simulink model "SensorFaultInj"  (R2013a)
settings: Solver=FixedStepDiscrete  SolverMode=SingleTasking  StartTime=0.0  StopTime=SimLength  FixedStep=SampleTime  RelTol=1e-3
values from neighbouring files (symbols this model uses):
  GlobalSeed = 10    [start_framework07.m]
  SampleTime = 0.01    [start_framework07.m]
  SimLength = 40    [start_framework07.m]
undefined symbols (not defined in the file or in its folder): DiscIntNeverNeededParam
libraries: dspswit3 x48, simulink x32
(part 3 of 9)

== system SensorFaultInj/FIM_Muster1/occurrence1/flank to dlock2 ==
  flank : Inport
  delay : Inport  Port=2
  Constant : Constant
  Constant1 : Constant  Value=0
  Counter2 : dspswit3/Counter  Direction=Up  CountEvent=Rising edge  CounterSize=User defined  MaxCount=512  InitialCount=0  Output=Count and Hit  HitValue=1  ResetInput=on  SamplesPerFrame=1  Ts=-1  CntDtype=double  HitDtype=Boolean
  Switch : Switch  Criteria=u2 > Threshold
  Variable Time Delay : VariableTransportDelay  MaximumDelay=512  ZeroDelay=on
  conv0 : DataTypeConversion  OutDataTypeStr=boolean
  conv1 : DataTypeConversion  OutDataTypeStr=double
  flag1 : Switch  Threshold=1
  block : Outport
  wires:
  Constant/1 -> flag1/1, Switch/1
  Constant1/1 -> Switch/3, flag1/3
  flank/1 -> Switch/2
  Switch/1 -> Counter2/1
  Counter2/1 -> flag1/2
  delay/1 -> Variable Time Delay/2
  Variable Time Delay/1 -> conv0/1
  flag1/1 -> block/1
  conv0/1 -> Counter2/2
  Counter2/2 -> conv1/1
  conv1/1 -> Variable Time Delay/1

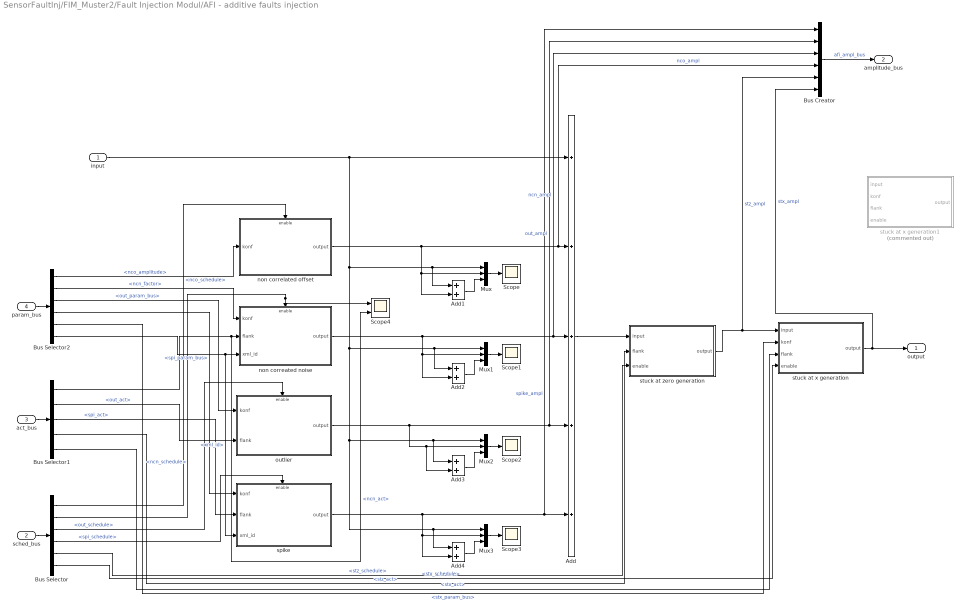
== system SensorFaultInj/FIM_Muster2/Fault Injection Modul/AFI - additive faults injection ==
  input : Inport
  sched_bus : Inport  Port=2
  act_bus : Inport  Port=3
  param_bus : Inport  Port=4
  Add : Sum  Inputs=+++++
  Add{1..4} (4 alike) : Sum
  Bus Creator : BusCreator  Inputs=6
  Bus Selector : BusSelector  OutputSignals=nco_schedule,ncn_schedule,out_schedule,spi_schedule,stz_schedule,stx_schedule
  Bus Selector1 : BusSelector  OutputSignals=ncn_act,out_act,spi_act,stz_act,stx_act
  Bus Selector2 : BusSelector  OutputSignals=nco_amplitude,ncn_factor,out_param_bus,spi_param_bus,stx_param_bus,xml_id
  Mux{,1..3} (4 alike) : Mux  Inputs=3
  Scope{,1..3} (4 alike) : Scope
      Scope settings: YMin=-70  YMax=70  SaveName=ScopeData14  MaxDataPoints=10000
      Scope1 settings: YMin=-50  YMax=55  SaveName=ScopeData15
      Scope2 settings: YMin=-70  YMax=70  SaveName=ScopeData16
      Scope3 settings: YMin=-50  YMax=60  SaveName=ScopeData17
  Scope4 : Scope  NumInputPorts=2
      settings: YMin=-70~-5  YMax=70~5  SaveName=ScopeData28
  non correated noise : Subsystem
  non correlated offset : Subsystem
  outlier : Subsystem
  spike : Subsystem
  stuck at x generation : Subsystem
  stuck at x generation1 : Subsystem  Commented=on
  stuck at zero generation : Subsystem
  output : Outport
  "amplitude_bus " : Outport  Port=2
  wires:
  input/1 -> Add1/1, Mux/1, Add4/1, Mux3/1, Add3/1, Mux2/1, Add2/1, Mux1/1, Add/1
  non correlated offset/1(output) -> Add1/2, Mux/2, Bus Creator/4, Add/2  "nco_ampl"
  non correated noise/1(output) -> Add2/2, Mux1/2, Bus Creator/3, Add/3  "ncn_ampl"
  outlier/1(output) -> Add3/2, Mux2/2, Bus Creator/2, Add/4  "out_ampl"
  spike/1(output) -> Bus Creator/1, Add/5, Add4/2, Mux3/2  "spike_ampl"
  Mux/1 -> Scope/1
  Mux1/1 -> Scope1/1
  Mux2/1 -> Scope2/1
  Mux3/1 -> Scope3/1
  Add1/1 -> Mux/3
  Add2/1 -> Mux1/3
  Add3/1 -> Mux2/3
  Add4/1 -> Mux3/3
  Add/1 -> stuck at zero generation/1(input)
  stuck at x generation/1(output) -> Bus Creator/6, output/1  "stx_ampl"
  stuck at zero generation/1(output) -> Bus Creator/5, stuck at x generation/1(input)  "stz_ampl"
  sched_bus/1 -> Bus Selector/1
  Bus Selector/1 -> non correlated offset/Enable  "<nco_schedule>"
  Bus Selector/2 -> Scope4/1, non correated noise/Enable  "<ncn_schedule>"
  Bus Selector/5 -> stuck at zero generation/3(enable)  "<stz_schedule>"
  Bus Selector/6 -> stuck at x generation/4(enable)  "<stx_schedule>"
  act_bus/1 -> Bus Selector1/1
  Bus Selector1/1 -> Scope4/2, non correated noise/2(flank)  "<ncn_act>"
  Bus Selector1/2 -> outlier/2(flank)  "<out_act>"
  Bus Selector1/3 -> spike/2(flank)  "<spi_act>"
  Bus Selector1/4 -> stuck at zero generation/2(flank)  "<stz_act>"
  Bus Selector1/5 -> stuck at x generation/3(flank)  "<stx_act>"
  param_bus/1 -> Bus Selector2/1
  Bus Selector2/1 -> non correlated offset/1(konf)  "<nco_amplitude>"
  Bus Selector2/2 -> non correated noise/1("konf ")  "<ncn_factor>"
  Bus Selector2/3 -> outlier/1(konf)  "<out_param_bus>"
  Bus Selector2/4 -> spike/1(konf)  "<spi_param_bus>"
  Bus Selector2/5 -> stuck at x generation/2(konf)  "<stx_param_bus>"
  Bus Selector2/6 -> spike/3(xml_id), non correated noise/3(xml_id)  "<xml_id>"
  Bus Creator/1 -> "amplitude_bus "/1  "afi_ampl_bus"
  Bus Selector/3 -> outlier/Enable  "<out_schedule>"
  Bus Selector/4 -> spike/Enable  "<spi_schedule>"

== system SensorFaultInj/FIM_Muster2/Fault Injection Modul/FFI - functional fault injection ==
  input : Inport
  schedule_port : Inport  Port=2
  param_port : Inport  Port=3
  Bus Creator : BusCreator  Inputs=3
  Bus Selector : BusSelector  OutputSignals=sat_schedule,ncd_schedule,tcd_schedule
  Bus Selector1 : BusSelector  OutputSignals=sat_param_bus,ncd_delay,tcd_delay,xml_id
  Mux1 : Mux  Inputs=2
  Mux3 : Mux  Inputs=3
  Scope3 : Scope  NumInputPorts=2
      settings: YMin=-50~-50  YMax=50~50  SaveName=ScopeData6
  "const delay " : Subsystem
  saturation : Subsystem
  "time correlated delay " : Subsystem
  output : Outport
  amplitude_port : Outport  Port=2
  wires:
  input/1 -> Mux3/1, Mux1/1, saturation/1(input)
  Mux1/1 -> Scope3/1
  Mux3/1 -> Scope3/2
  saturation/1(output) -> Mux1/2, Bus Creator/1, "const delay "/1(input)  "sat_ampl"
  "const delay "/1(output1) -> "time correlated delay "/1(input), Mux3/2
  "time correlated delay "/1(output1) -> Mux3/3, output/1
  schedule_port/1 -> Bus Selector/1
  param_port/1 -> Bus Selector1/1
  Bus Selector1/4 -> "time correlated delay "/4(xml id)  "<xml_id>"
  Bus Selector1/3 -> "time correlated delay "/2(konf)  "<tcd_delay>"
  Bus Selector1/1 -> saturation/2("konf ")  "<sat_param_bus>"
  Bus Selector1/2 -> "const delay "/2(konf)  "<ncd_delay>"
  Bus Selector/1 -> saturation/3(enable)  "<sat_schedule>"
  Bus Selector/2 -> "const delay "/3(enable)  "<ncd_schedule>"
  Bus Selector/3 -> "time correlated delay "/3(enable)  "<tcd_schedule>"
  Bus Creator/1 -> amplitude_port/1  "ffi_ampl_bus"
  "const delay "/2(delay) -> Bus Creator/2  "ncd_ampl"
  "time correlated delay "/2(delay) -> Bus Creator/3  "tcd_ampl"

== system SensorFaultInj/FIM_Muster2/Fault Injection Modul/MFI - multiplicative fault injection ==
  In1 : Inport
  sched_port : Inport  Port=2
  act_port : Inport  Port=3
  param_port : Inport  Port=4
  Add : Sum  Inputs=+++++
  Add{1..4} (4 alike) : Sum
  Bus Creator : BusCreator
  Bus Selector : BusSelector  OutputSignals=vco_schedule,tco_schedule,vcn_schedule,tcn_schedule
  Bus Selector1 : BusSelector  OutputSignals=vcn_act,tcn_act
  Bus Selector2 : BusSelector  OutputSignals=vco_factor,tco_amplitude,vcn_factor,tcn_factor,xml_id
  Mux{,1..3} (4 alike) : Mux  Inputs=3
  Scope{,1..3} (4 alike) : Scope
      Scope settings: YMin=-55  YMax=55  SaveName=ScopeData8
      Scope1 settings: YMin=-50  YMax=55  SaveName=ScopeData11  MaxDataPoints=10000
      Scope2 settings: YMin=-70  YMax=70  SaveName=ScopeData12
      Scope3 settings: YMin=-50  YMax=60  SaveName=ScopeData13
  time correlated noise : Subsystem  TreatAsAtomicUnit=on
  time correlated offset : Subsystem  TreatAsAtomicUnit=on
  value correlated noise : Subsystem
  value correlated offset : Subsystem  TreatAsAtomicUnit=on
  output : Outport
  "amplitude_port " : Outport  Port=2
  wires:
  In1/1 -> Mux3/1, Add4/1, Mux2/1, Add3/1, Mux1/1, Add2/1, Mux/1, Add1/1, Add/1, value correlated noise/1(input), value correlated offset/1(input)
  value correlated offset/1(output) -> Bus Creator/4, Add/2, Add1/2, Mux/2  "vco_ampl"
  time correlated offset/1(output) -> Add2/2, Mux1/2, Bus Creator/3, Add/3  "tco_ampl"
  value correlated noise/1(output) -> Add3/2, Mux2/2, Bus Creator/2, Add/4  "vcn_ampl"
  time correlated noise/1(output) -> Add4/2, Mux3/2, Bus Creator/1, Add/5  "tcn_ampl"
  Mux/1 -> Scope/1
  Mux1/1 -> Scope1/1
  Mux2/1 -> Scope2/1
  Mux3/1 -> Scope3/1
  Add1/1 -> Mux/3
  Add2/1 -> Mux1/3
  Add3/1 -> Mux2/3
  Add4/1 -> Mux3/3
  Add/1 -> output/1
  sched_port/1 -> Bus Selector/1
  Bus Selector/1 -> value correlated offset/Enable  "<vco_schedule>"
  Bus Selector/2 -> time correlated offset/Enable  "<tco_schedule>"
  Bus Selector/3 -> value correlated noise/Enable  "<vcn_schedule>"
  Bus Selector/4 -> time correlated noise/Enable  "<tcn_schedule>"
  act_port/1 -> Bus Selector1/1
  Bus Selector1/2 -> time correlated noise/2(flank)  "<tcn_act>"
  Bus Selector1/1 -> value correlated noise/3(flank)  "<vcn_act>"
  param_port/1 -> Bus Selector2/1
  Bus Selector2/5 -> value correlated noise/4(xml_id), time correlated noise/3(xml id), time correlated offset/2(xml id)  "<xml_id>"
  Bus Selector2/1 -> value correlated offset/2(konf)  "<vco_factor>"
  Bus Selector2/2 -> time correlated offset/1(konf)  "<tco_amplitude>"
  Bus Selector2/3 -> value correlated noise/2(konf)  "<vcn_factor>"
  Bus Selector2/4 -> time correlated noise/1(konf)  "<tcn_factor>"
  Bus Creator/1 -> "amplitude_port "/1  "mfi_amp_bus"

== system SensorFaultInj/FIM_Muster2/Fault Injection Modul/activation bus creator ==
  act_port : Inport
  Bus Selector : BusSelector  OutputSignals=vcn_act,tcn_act  OutputAsBus=on
  Bus Selector1 : BusSelector  OutputSignals=ncn_act,out_act,spi_act,stz_act,stx_act  OutputAsBus=on
  mfi_act_port : Outport
  afi_act_port : Outport  Port=2
  wires:
  act_port/1 -> Bus Selector1/1, Bus Selector/1
  Bus Selector/1 -> mfi_act_port/1  "mfi_act_bus"
  Bus Selector1/1 -> afi_act_port/1  "afi_act_bus"

== system SensorFaultInj/FIM_Muster2/Fault Injection Modul/schedule bus creator ==
  schedule_port : Inport
  Bus Selector : BusSelector  OutputSignals=vco_schedule,tco_schedule,vcn_schedule,tcn_schedule  OutputAsBus=on
  Bus Selector1 : BusSelector  OutputSignals=nco_schedule,ncn_schedule,spi_schedule,out_schedule,stz_schedule,stx_schedule  OutputAsBus=on
  Bus Selector2 : BusSelector  OutputSignals=sat_schedule,ncd_schedule,tcd_schedule  OutputAsBus=on
  mfi_sched_port : Outport
  afi_sched_port : Outport  Port=2
  ffi_sched_port : Outport  Port=3
  wires:
  schedule_port/1 -> Bus Selector2/1, Bus Selector1/1, Bus Selector/1
  Bus Selector/1 -> mfi_sched_port/1  "mfi_sched_bus"
  Bus Selector1/1 -> afi_sched_port/1  "afi_sched_bus"
  Bus Selector2/1 -> ffi_sched_port/1  "ffi_sched_bus"

== system SensorFaultInj/FIM_Muster2/Fault Injection Modul/schedule bus creator1 ==
  schedule_port : Inport
  Bus Selector : BusSelector  OutputSignals=parameter_bus.vco_factor,parameter_bus.tco_amplitude,parameter_bus.vcn_factor,parameter_bus.tcn_factor,xml_id  OutputAsBus=on
  Bus Selector1 : BusSelector  OutputSignals=parameter_bus.nco_amplitude,parameter_bus.ncn_factor,parameter_bus.out_param_bus,parameter_bus.spi_param_bus,parameter_bus.stx_param_bus,xml_id  OutputAsBus=on
  Bus Selector2 : BusSelector  OutputSignals=parameter_bus.sat_param_bus,parameter_bus.ncd_delay,parameter_bus.tcd_delay,xml_id  OutputAsBus=on
  mfi_sched_port : Outport
  afi_sched_port : Outport  Port=2
  ffi_sched_port : Outport  Port=3
  wires:
  schedule_port/1 -> Bus Selector2/1, Bus Selector1/1, Bus Selector/1
  Bus Selector/1 -> mfi_sched_port/1  "mfi_sched_bus"
  Bus Selector1/1 -> afi_sched_port/1  "afi_sched_bus"
  Bus Selector2/1 -> ffi_sched_port/1  "ffi_sched_bus"

== system SensorFaultInj/FIM_Muster2/Parser Modul/occurence parser  ==
  In1 : Inport
  Add1 : Sum
  Constant1 : Constant
  Digital Clock2 : DigitalClock  SampleTime=SampleTime
  Enabled Subsystem : Subsystem  TreatAsAtomicUnit=on
  Memory2 : Memory
  Subtract2 : Sum  Inputs=+-
  Out1 : Outport
  wires:
  Digital Clock2/1 -> Add1/2
  Memory2/1 -> Subtract2/2
  Constant1/1 -> Add1/1, Subtract2/1
  Add1/1 -> Memory2/1
  Subtract2/1 -> Enabled Subsystem/Enable
  Enabled Subsystem/1(Out1) -> Out1/1
  In1/1 -> Enabled Subsystem/1(In1)

== system SensorFaultInj/FIM_Muster2/Parser Modul/parameter parser ==
  In1 : Inport
  Add1 : Sum
  Constant1 : Constant
  Digital Clock2 : DigitalClock  SampleTime=SampleTime
  Enabled Subsystem : Subsystem  TreatAsAtomicUnit=on
  Memory2 : Memory
  Subtract2 : Sum  Inputs=+-
  Out1 : Outport
  wires:
  Digital Clock2/1 -> Add1/2
  Memory2/1 -> Subtract2/2
  Constant1/1 -> Add1/1, Subtract2/1
  Add1/1 -> Memory2/1
  Subtract2/1 -> Enabled Subsystem/Enable
  In1/1 -> Enabled Subsystem/1(In1)
  Enabled Subsystem/1(Out1) -> Out1/1

== system SensorFaultInj/FIM_Muster2/Parser Modul/schedule once per sample step  ==
  In1 : Inport
  Bus Creator : BusCreator  Inputs=13
  schedule_fcn id 0 : Subsystem
  schedule_fcn id 1 : Subsystem
  schedule_fcn id 10 : Subsystem
  schedule_fcn id 11 : Subsystem
  schedule_fcn id 12 : Subsystem
  schedule_fcn id 2 : Subsystem
  schedule_fcn id 3 : Subsystem
  schedule_fcn id 4 : Subsystem
  schedule_fcn id 5 : Subsystem
  schedule_fcn id 6 : Subsystem
  schedule_fcn id 7 : Subsystem
  schedule_fcn id 8 : Subsystem
  schedule_fcn id 9 : Subsystem
  Out1 : Outport
  wires:
  schedule_fcn id 3/1(output) -> Bus Creator/4
  schedule_fcn id 6/1(output) -> Bus Creator/7
  schedule_fcn id 4/1(output) -> Bus Creator/5
  schedule_fcn id 1/1(output) -> Bus Creator/2
  schedule_fcn id 0/1(output) -> Bus Creator/1
  schedule_fcn id 10/1(output) -> Bus Creator/11
  schedule_fcn id 5/1(output) -> Bus Creator/6
  schedule_fcn id 9/1(output) -> Bus Creator/10
  schedule_fcn id 8/1(output) -> Bus Creator/9
  schedule_fcn id 7/1(output) -> Bus Creator/8
  schedule_fcn id 12/1(output) -> Bus Creator/13
  schedule_fcn id 11/1(output) -> Bus Creator/12
  schedule_fcn id 2/1(output) -> Bus Creator/3
  Bus Creator/1 -> Out1/1  "schedule_bus"
  In1/1 -> schedule_fcn id 5/1(In1), schedule_fcn id 4/1(In1), schedule_fcn id 3/1(In1), schedule_fcn id 2/1(In1), schedule_fcn id 1/1(In1), schedule_fcn id 0/1(In1), schedule_fcn id 6/1(In1), schedule_fcn id 7/1(In1), schedule_fcn id 8/1(In1), schedule_fcn id 9/1(In1), schedule_fcn id 10/1(In1), schedule_fcn id 12/1(In1), schedule_fcn id 11/1(In1)

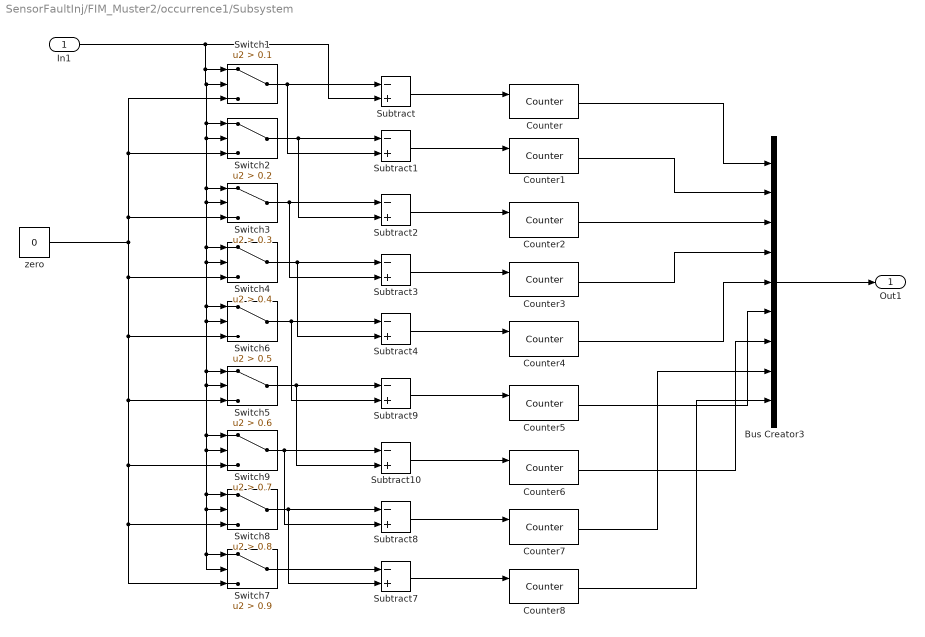
== system SensorFaultInj/FIM_Muster2/occurrence1/Subsystem ==
  In1 : Inport
  Bus Creator3 : BusCreator  Inputs=9
  Counter{,1..8} (9 alike) : dspswit3/Counter  Direction=Up  CountEvent=Non-zero sample  CounterSize=User defined  MaxCount=10000  InitialCount=0  Output=Count  HitValue=32  ResetInput=on  SamplesPerFrame=1  Ts=1  CntDtype=double  HitDtype=Logical
  Subtract{,1..4,7..10} (9 alike) : Sum  Inputs=-+
  Switch1 : Switch  Criteria=u2 > Threshold  Threshold=0.1
  Switch2 : Switch  Criteria=u2 > Threshold  Threshold=0.2
  Switch3 : Switch  Criteria=u2 > Threshold  Threshold=0.3
  Switch4 : Switch  Criteria=u2 > Threshold  Threshold=0.4
  Switch5 : Switch  Criteria=u2 > Threshold  Threshold=0.6
  Switch6 : Switch  Criteria=u2 > Threshold  Threshold=0.5
  Switch7 : Switch  Criteria=u2 > Threshold  Threshold=0.9
  Switch8 : Switch  Criteria=u2 > Threshold  Threshold=0.8
  Switch9 : Switch  Criteria=u2 > Threshold  Threshold=0.7
  zero : Constant  Value=0  OutDataTypeStr=boolean
  Out1 : Outport
  wires:
  Switch1/1 -> Subtract1/2, Subtract/1
  Switch2/1 -> Subtract2/2, Subtract1/1
  Switch3/1 -> Subtract3/2, Subtract2/1
  Switch4/1 -> Subtract4/2, Subtract3/1
  Switch6/1 -> Subtract9/2, Subtract4/1
  Switch5/1 -> Subtract10/2, Subtract9/1
  Switch9/1 -> Subtract8/2, Subtract10/1
  Switch8/1 -> Subtract7/2, Subtract8/1
  Switch7/1 -> Subtract7/1
  Subtract/1 -> Counter/1
  Subtract1/1 -> Counter1/1
  Subtract2/1 -> Counter2/1
  Subtract3/1 -> Counter3/1
  Subtract4/1 -> Counter4/1
  Subtract9/1 -> Counter5/1
  Subtract10/1 -> Counter6/1
  Subtract8/1 -> Counter7/1
  Counter2/1 -> Bus Creator3/3
  Counter3/1 -> Bus Creator3/4
  Counter1/1 -> Bus Creator3/2
  Counter/1 -> Bus Creator3/1
  Counter4/1 -> Bus Creator3/5
  Counter5/1 -> Bus Creator3/6
  Counter6/1 -> Bus Creator3/7
  Counter7/1 -> Bus Creator3/8
  Counter8/1 -> Bus Creator3/9
  Bus Creator3/1 -> Out1/1
  In1/1 -> Switch2/1, Switch3/1, Switch3/2, Switch4/1, Switch4/2, Switch6/1, Switch5/1, Switch9/1, Switch8/1, Switch7/1, Switch7/2, Switch8/2, Switch9/2, Switch5/2, Switch6/2, Switch2/2, Switch1/2, Switch1/1, Subtract/2
  zero/1 -> Switch4/3, Switch6/3, Switch5/3, Switch9/3, Switch7/3, Switch8/3, Switch1/3, Switch2/3, Switch3/3
  Subtract7/1 -> Counter8/1

== system SensorFaultInj/FIM_Muster2/occurrence1/bus_counter ==
  In1 : Inport
  Bus Creator : BusCreator  Inputs=7
  Bus Selector : BusSelector  OutputSignals=vcn_act,tcn_act,ncn_act,out_act,spi_act,stz_act,stx_act
  Counter{,1..3} (4 alike) : dspswit3/Counter  Direction=Up  CountEvent=Non-zero sample  CounterSize=User defined  MaxCount=10000  InitialCount=0  Output=Count  HitValue=32  ResetInput=on  SamplesPerFrame=1  Ts=1  CntDtype=double  HitDtype=Logical
  Counter4 : dspswit3/Counter  Direction=Up  CountEvent=Rising edge  CounterSize=User defined  MaxCount=10000  InitialCount=0  Output=Count  HitValue=32  ResetInput=on  SamplesPerFrame=1  Ts=1  CntDtype=double  HitDtype=Logical
  Counter5 : dspswit3/Counter  Direction=Up  CountEvent=Rising edge  CounterSize=User defined  MaxCount=10000  InitialCount=0  Output=Count  HitValue=32  ResetInput=on  SamplesPerFrame=1  Ts=1  CntDtype=double  HitDtype=Logical
  Counter6 : dspswit3/Counter  Direction=Up  CountEvent=Rising edge  CounterSize=User defined  MaxCount=10000  InitialCount=0  Output=Count  HitValue=32  ResetInput=on  SamplesPerFrame=1  Ts=1  CntDtype=double  HitDtype=Logical
  Out1 : Outport
  wires:
  In1/1 -> Bus Selector/1
  Bus Selector/1 -> Counter/1  "<vcn_act>"
  Counter/1 -> Bus Creator/1
  Counter1/1 -> Bus Creator/2
  Bus Selector/2 -> Counter1/1  "<tcn_act>"
  Bus Selector/3 -> Counter2/1  "<ncn_act>"
  Bus Selector/4 -> Counter3/1  "<out_act>"
  Bus Selector/5 -> Counter4/1  "<spi_act>"
  Bus Selector/6 -> Counter5/1  "<stz_act>"
  Bus Selector/7 -> Counter6/1  "<stx_act>"
  Counter3/1 -> Bus Creator/4
  Counter4/1 -> Bus Creator/5
  Counter6/1 -> Bus Creator/7
  Counter5/1 -> Bus Creator/6
  Counter2/1 -> Bus Creator/3
  Bus Creator/1 -> Out1/1

== system SensorFaultInj/FIM_Muster2/occurrence1/disable non active trigger ==
  vec_probability : Inport
  vec_activation : Inport  Port=2
  Bus Creator : BusCreator  Inputs=7
  Bus Selector : BusSelector  OutputSignals=vcn_occ,tcn_occ,ncn_occ,out_occ,spi_occ,stz_occ,stx_occ
  Bus Selector1 : BusSelector  OutputSignals=vcn_schedule,tcn_schedule,ncn_schedule,out_schedule,spi_schedule,stz_schedule,stx_schedule
  Constant : Constant  Value=0
  Switch{,1..6} (7 alike) : Switch  Threshold=1
  vec_probability_ad : Outport
  wires:
  vec_probability/1 -> Bus Selector/1
  vec_activation/1 -> Bus Selector1/1
  Bus Selector1/1 -> Switch/2  "<vcn_schedule>"
  Bus Selector1/2 -> Switch1/2  "<tcn_schedule>"
  Bus Selector1/3 -> Switch2/2  "<ncn_schedule>"
  Bus Selector1/4 -> Switch3/2  "<out_schedule>"
  Bus Selector1/5 -> Switch6/2  "<spi_schedule>"
  Bus Selector1/6 -> Switch5/2  "<stz_schedule>"
  Bus Selector1/7 -> Switch4/2  "<stx_schedule>"
  Bus Selector/1 -> Switch/1  "<vcn_occ>"
  Bus Selector/2 -> Switch1/1  "<tcn_occ>"
  Bus Selector/3 -> Switch2/1  "<ncn_occ>"
  Bus Selector/4 -> Switch3/1  "<out_occ>"
  Bus Selector/5 -> Switch6/1  "<spi_occ>"
  Constant/1 -> Switch4/3, Switch5/3, Switch6/3, Switch3/3, Switch2/3, Switch1/3, Switch/3
  Switch/1 -> Bus Creator/1  "vcn_occ"
  Switch1/1 -> Bus Creator/2  "tcn_occ"
  Switch2/1 -> Bus Creator/3  "ncn_occ"
  Switch3/1 -> Bus Creator/4  "out_occ"
  Switch6/1 -> Bus Creator/5  "spi_occ"
  Switch5/1 -> Bus Creator/6  "stz_occ"
  Switch4/1 -> Bus Creator/7  "stx_occ"
  Bus Selector/7 -> Switch4/1  "<stx_occ>"
  Bus Selector/6 -> Switch5/1  "<stz_occ>"
  Bus Creator/1 -> vec_probability_ad/1

== system SensorFaultInj/FIM_Muster2/occurrence1/flank to dlock0 ==
  flank : Inport
  delay : Inport  Port=2
  Constant : Constant
  Constant1 : Constant  Value=0
  Counter2 : dspswit3/Counter  Direction=Up  CountEvent=Rising edge  CounterSize=User defined  MaxCount=512  InitialCount=0  Output=Count and Hit  HitValue=1  ResetInput=on  SamplesPerFrame=1  Ts=-1  CntDtype=double  HitDtype=Boolean
  Switch : Switch  Criteria=u2 > Threshold
  Variable Time Delay : VariableTransportDelay  MaximumDelay=512  ZeroDelay=on
  conv0 : DataTypeConversion  OutDataTypeStr=boolean
  conv1 : DataTypeConversion  OutDataTypeStr=double
  flag1 : Switch  Threshold=1
  block : Outport
  wires:
  Constant/1 -> flag1/1, Switch/1
  Constant1/1 -> Switch/3, flag1/3
  flank/1 -> Switch/2
  Switch/1 -> Counter2/1
  Counter2/1 -> flag1/2
  delay/1 -> Variable Time Delay/2
  Variable Time Delay/1 -> conv0/1
  flag1/1 -> block/1
  conv0/1 -> Counter2/2
  Counter2/2 -> conv1/1
  conv1/1 -> Variable Time Delay/1

== system SensorFaultInj/FIM_Muster2/occurrence1/flank to dlock1 ==
  flank : Inport
  delay : Inport  Port=2
  Constant : Constant
  Constant1 : Constant  Value=0
  Counter2 : dspswit3/Counter  Direction=Up  CountEvent=Rising edge  CounterSize=User defined  MaxCount=512  InitialCount=0  Output=Count and Hit  HitValue=1  ResetInput=on  SamplesPerFrame=1  Ts=-1  CntDtype=double  HitDtype=Boolean
  Switch : Switch  Criteria=u2 > Threshold
  Variable Time Delay : VariableTransportDelay  MaximumDelay=512  ZeroDelay=on
  conv0 : DataTypeConversion  OutDataTypeStr=boolean
  conv1 : DataTypeConversion  OutDataTypeStr=double
  flag1 : Switch  Threshold=1
  block : Outport
  wires:
  Constant/1 -> flag1/1, Switch/1
  Constant1/1 -> Switch/3, flag1/3
  flank/1 -> Switch/2
  Switch/1 -> Counter2/1
  Counter2/1 -> flag1/2
  delay/1 -> Variable Time Delay/2
  Variable Time Delay/1 -> conv0/1
  flag1/1 -> block/1
  conv0/1 -> Counter2/2
  Counter2/2 -> conv1/1
  conv1/1 -> Variable Time Delay/1

== system SensorFaultInj/FIM_Muster2/occurrence1/flank to dlock2 ==
  flank : Inport
  delay : Inport  Port=2
  Constant : Constant
  Constant1 : Constant  Value=0
  Counter2 : dspswit3/Counter  Direction=Up  CountEvent=Rising edge  CounterSize=User defined  MaxCount=512  InitialCount=0  Output=Count and Hit  HitValue=1  ResetInput=on  SamplesPerFrame=1  Ts=-1  CntDtype=double  HitDtype=Boolean
  Switch : Switch  Criteria=u2 > Threshold
  Variable Time Delay : VariableTransportDelay  MaximumDelay=512  ZeroDelay=on
  conv0 : DataTypeConversion  OutDataTypeStr=boolean
  conv1 : DataTypeConversion  OutDataTypeStr=double
  flag1 : Switch  Threshold=1
  block : Outport
  wires:
  Constant/1 -> flag1/1, Switch/1
  Constant1/1 -> Switch/3, flag1/3
  flank/1 -> Switch/2
  Switch/1 -> Counter2/1
  Counter2/1 -> flag1/2
  delay/1 -> Variable Time Delay/2
  Variable Time Delay/1 -> conv0/1
  flag1/1 -> block/1
  conv0/1 -> Counter2/2
  Counter2/2 -> conv1/1
  conv1/1 -> Variable Time Delay/1

== system SensorFaultInj/Glogal Activation Generator/Enabled Subsystem/global parser2 ==
  ex_sfun_globalocc : S-Function  FunctionName=ex_sfun_globalocc  EnableBusSupport=off  mask(Legacy Function){SFunctionSpec=double y1 = global_occ(single u1), ShowSpec=on}
      mask prompts: ShowSpec "Display function specification"
      mask help:
      | This block allows you to call the legacy functions specified by the following Legacy Code Tool definition:
      | def.SFunctionName = 'ex_sfun_globalocc';
      | def.OutputFcnSpec = 'double y1 = global_occ(single u1)';
      | def.HeaderFiles = {'global_occ.hpp'};
      | def.SourceFiles = {'global_occ.cpp'};
      | def.Options.language = 'C++';
      mask Help: <p>This block was generated automatically by the Legacy Code Tool. For detailed help on this tool, call<a href="matlab:legacy_code('help')"> legacy_code('help')</a>.</p>
      mask Callback ShowSpec:
      | if strcmp(get_param(gcbh, 'ShowSpec'), 'on')
      |   set_param(gcbh, 'MaskDisplay', sprintf('fprintf(''%s'');', get_param(gcbh, 'SFunctionSpec')));
      | else
      |   set_param(gcbh, 'MaskDisplay', sprintf('fprintf(''%s'');', get_param(gcbh, 'FunctionName')));
      | end
      mask Display: fprintf('double y1 = global_occ(single u1)');
  fault id : Constant  Value=2  OutDataTypeStr=single
  occ : Outport
  wires:
  ex_sfun_globalocc/1 -> occ/1  "glo_vcn_occ"
  fault id/1 -> ex_sfun_globalocc/1

== system SensorFaultInj/Glogal Activation Generator/Enabled Subsystem/global parser3 ==
  ex_sfun_globalocc : S-Function  FunctionName=ex_sfun_globalocc  EnableBusSupport=off  mask(Legacy Function){SFunctionSpec=double y1 = global_occ(single u1), ShowSpec=on}
      mask prompts: ShowSpec "Display function specification"
      mask help:
      | This block allows you to call the legacy functions specified by the following Legacy Code Tool definition:
      | def.SFunctionName = 'ex_sfun_globalocc';
      | def.OutputFcnSpec = 'double y1 = global_occ(single u1)';
      | def.HeaderFiles = {'global_occ.hpp'};
      | def.SourceFiles = {'global_occ.cpp'};
      | def.Options.language = 'C++';
      mask Help: <p>This block was generated automatically by the Legacy Code Tool. For detailed help on this tool, call<a href="matlab:legacy_code('help')"> legacy_code('help')</a>.</p>
      mask Callback ShowSpec:
      | if strcmp(get_param(gcbh, 'ShowSpec'), 'on')
      |   set_param(gcbh, 'MaskDisplay', sprintf('fprintf(''%s'');', get_param(gcbh, 'SFunctionSpec')));
      | else
      |   set_param(gcbh, 'MaskDisplay', sprintf('fprintf(''%s'');', get_param(gcbh, 'FunctionName')));
      | end
      mask Display: fprintf('double y1 = global_occ(single u1)');
  fault id : Constant  Value=3  OutDataTypeStr=single
  occ : Outport
  wires:
  ex_sfun_globalocc/1 -> occ/1  "glo_tcn_occ"
  fault id/1 -> ex_sfun_globalocc/1

== system SensorFaultInj/Glogal Activation Generator/Enabled Subsystem/global parser5 ==
  ex_sfun_globalocc : S-Function  FunctionName=ex_sfun_globalocc  EnableBusSupport=off  mask(Legacy Function){SFunctionSpec=double y1 = global_occ(single u1), ShowSpec=on}
      mask prompts: ShowSpec "Display function specification"
      mask help:
      | This block allows you to call the legacy functions specified by the following Legacy Code Tool definition:
      | def.SFunctionName = 'ex_sfun_globalocc';
      | def.OutputFcnSpec = 'double y1 = global_occ(single u1)';
      | def.HeaderFiles = {'global_occ.hpp'};
      | def.SourceFiles = {'global_occ.cpp'};
      | def.Options.language = 'C++';
      mask Help: <p>This block was generated automatically by the Legacy Code Tool. For detailed help on this tool, call<a href="matlab:legacy_code('help')"> legacy_code('help')</a>.</p>
      mask Callback ShowSpec:
      | if strcmp(get_param(gcbh, 'ShowSpec'), 'on')
      |   set_param(gcbh, 'MaskDisplay', sprintf('fprintf(''%s'');', get_param(gcbh, 'SFunctionSpec')));
      | else
      |   set_param(gcbh, 'MaskDisplay', sprintf('fprintf(''%s'');', get_param(gcbh, 'FunctionName')));
      | end
      mask Display: fprintf('double y1 = global_occ(single u1)');
  fault id : Constant  Value=5  OutDataTypeStr=single
  occ : Outport
  wires:
  ex_sfun_globalocc/1 -> occ/1  "glo_ncn_occ"
  fault id/1 -> ex_sfun_globalocc/1

== system SensorFaultInj/Glogal Activation Generator/Enabled Subsystem/global parser6 ==
  ex_sfun_globalocc : S-Function  FunctionName=ex_sfun_globalocc  EnableBusSupport=off  mask(Legacy Function){SFunctionSpec=double y1 = global_occ(single u1), ShowSpec=on}
      mask prompts: ShowSpec "Display function specification"
      mask help:
      | This block allows you to call the legacy functions specified by the following Legacy Code Tool definition:
      | def.SFunctionName = 'ex_sfun_globalocc';
      | def.OutputFcnSpec = 'double y1 = global_occ(single u1)';
      | def.HeaderFiles = {'global_occ.hpp'};
      | def.SourceFiles = {'global_occ.cpp'};
      | def.Options.language = 'C++';
      mask Help: <p>This block was generated automatically by the Legacy Code Tool. For detailed help on this tool, call<a href="matlab:legacy_code('help')"> legacy_code('help')</a>.</p>
      mask Callback ShowSpec:
      | if strcmp(get_param(gcbh, 'ShowSpec'), 'on')
      |   set_param(gcbh, 'MaskDisplay', sprintf('fprintf(''%s'');', get_param(gcbh, 'SFunctionSpec')));
      | else
      |   set_param(gcbh, 'MaskDisplay', sprintf('fprintf(''%s'');', get_param(gcbh, 'FunctionName')));
      | end
      mask Display: fprintf('double y1 = global_occ(single u1)');
  fault id : Constant  Value=6  OutDataTypeStr=single
  occ : Outport
  wires:
  ex_sfun_globalocc/1 -> occ/1  "glo_out_occ"
  fault id/1 -> ex_sfun_globalocc/1

== system SensorFaultInj/Glogal Activation Generator/Enabled Subsystem/global parser7 ==
  ex_sfun_globalocc : S-Function  FunctionName=ex_sfun_globalocc  EnableBusSupport=off  mask(Legacy Function){SFunctionSpec=double y1 = global_occ(single u1), ShowSpec=on}
      mask prompts: ShowSpec "Display function specification"
      mask help:
      | This block allows you to call the legacy functions specified by the following Legacy Code Tool definition:
      | def.SFunctionName = 'ex_sfun_globalocc';
      | def.OutputFcnSpec = 'double y1 = global_occ(single u1)';
      | def.HeaderFiles = {'global_occ.hpp'};
      | def.SourceFiles = {'global_occ.cpp'};
      | def.Options.language = 'C++';
      mask Help: <p>This block was generated automatically by the Legacy Code Tool. For detailed help on this tool, call<a href="matlab:legacy_code('help')"> legacy_code('help')</a>.</p>
      mask Callback ShowSpec:
      | if strcmp(get_param(gcbh, 'ShowSpec'), 'on')
      |   set_param(gcbh, 'MaskDisplay', sprintf('fprintf(''%s'');', get_param(gcbh, 'SFunctionSpec')));
      | else
      |   set_param(gcbh, 'MaskDisplay', sprintf('fprintf(''%s'');', get_param(gcbh, 'FunctionName')));
      | end
      mask Display: fprintf('double y1 = global_occ(single u1)');
  fault id : Constant  Value=7  OutDataTypeStr=single
  occ : Outport
  wires:
  ex_sfun_globalocc/1 -> occ/1  "glo_spi_occ"
  fault id/1 -> ex_sfun_globalocc/1

== system SensorFaultInj/Glogal Activation Generator/Enabled Subsystem/global parser8 ==
  ex_sfun_globalocc : S-Function  FunctionName=ex_sfun_globalocc  EnableBusSupport=off  mask(Legacy Function){SFunctionSpec=double y1 = global_occ(single u1), ShowSpec=on}
      mask prompts: ShowSpec "Display function specification"
      mask help:
      | This block allows you to call the legacy functions specified by the following Legacy Code Tool definition:
      | def.SFunctionName = 'ex_sfun_globalocc';
      | def.OutputFcnSpec = 'double y1 = global_occ(single u1)';
      | def.HeaderFiles = {'global_occ.hpp'};
      | def.SourceFiles = {'global_occ.cpp'};
      | def.Options.language = 'C++';
      mask Help: <p>This block was generated automatically by the Legacy Code Tool. For detailed help on this tool, call<a href="matlab:legacy_code('help')"> legacy_code('help')</a>.</p>
      mask Callback ShowSpec:
      | if strcmp(get_param(gcbh, 'ShowSpec'), 'on')
      |   set_param(gcbh, 'MaskDisplay', sprintf('fprintf(''%s'');', get_param(gcbh, 'SFunctionSpec')));
      | else
      |   set_param(gcbh, 'MaskDisplay', sprintf('fprintf(''%s'');', get_param(gcbh, 'FunctionName')));
      | end
      mask Display: fprintf('double y1 = global_occ(single u1)');
  fault id : Constant  Value=8  OutDataTypeStr=single
  occ : Outport
  wires:
  ex_sfun_globalocc/1 -> occ/1  "glo_stz_occ"
  fault id/1 -> ex_sfun_globalocc/1

== system SensorFaultInj/Glogal Activation Generator/Enabled Subsystem/global parser9 ==
  ex_sfun_globalocc : S-Function  FunctionName=ex_sfun_globalocc  EnableBusSupport=off  mask(Legacy Function){SFunctionSpec=double y1 = global_occ(single u1), ShowSpec=on}
      mask prompts: ShowSpec "Display function specification"
      mask help:
      | This block allows you to call the legacy functions specified by the following Legacy Code Tool definition:
      | def.SFunctionName = 'ex_sfun_globalocc';
      | def.OutputFcnSpec = 'double y1 = global_occ(single u1)';
      | def.HeaderFiles = {'global_occ.hpp'};
      | def.SourceFiles = {'global_occ.cpp'};
      | def.Options.language = 'C++';
      mask Help: <p>This block was generated automatically by the Legacy Code Tool. For detailed help on this tool, call<a href="matlab:legacy_code('help')"> legacy_code('help')</a>.</p>
      mask Callback ShowSpec:
      | if strcmp(get_param(gcbh, 'ShowSpec'), 'on')
      |   set_param(gcbh, 'MaskDisplay', sprintf('fprintf(''%s'');', get_param(gcbh, 'SFunctionSpec')));
      | else
      |   set_param(gcbh, 'MaskDisplay', sprintf('fprintf(''%s'');', get_param(gcbh, 'FunctionName')));
      | end
      mask Display: fprintf('double y1 = global_occ(single u1)');
  fault id : Constant  Value=9  OutDataTypeStr=single
  occ : Outport
  wires:
  ex_sfun_globalocc/1 -> occ/1  "glo_stx_occ"
  fault id/1 -> ex_sfun_globalocc/1

== system SensorFaultInj/FIM_Muster/Fault Injection Modul/AFI - additive faults injection/non correated noise ==
  "konf " : Inport
  flank : Inport  Port=2
  xml_id : Inport  Port=3
  Enable : EnablePort
  Product : Product
  Scope : Scope
      settings: SaveName=ScopeData4
  Switch : Switch  Threshold=1
  pdf_parser : Subsystem
  zero : Constant  Value=0
  output : Outport  OutputWhenDisabled=reset  InitialOutput=[0]
  wires:
  zero/1 -> Switch/3
  Switch/1 -> output/1
  flank/1 -> Switch/2
  pdf_parser/1(distr value) -> Product/1
  Product/1 -> Switch/1, Scope/1
  "konf "/1 -> Product/2
  xml_id/1 -> pdf_parser/1(xml id)

== system SensorFaultInj/FIM_Muster/Fault Injection Modul/AFI - additive faults injection/non correlated offset ==
  konf : Inport
  Enable : EnablePort
  output : Outport  OutputWhenDisabled=reset  InitialOutput=[0]
  wires:
  konf/1 -> output/1

== system SensorFaultInj/FIM_Muster/Fault Injection Modul/AFI - additive faults injection/outlier ==
  konf : Inport
  flank : Inport  Port=2
  Enable : EnablePort
  Add : Sum
  Bus Selector : BusSelector  OutputSignals=out_amplitude,out_neg
  Interpreted MATLAB Function : MATLABFcn  MATLABFcn=rand
  Interpreted MATLAB Function1 : MATLABFcn  Commented=on
  Product : Product
  Product1 : Product
  Product2 : Product
  Switch1 : Switch  Threshold=1
  Switch2 : Switch  Threshold=1
  const : Constant
  const1 : Constant  Value=-0.5
  const2 : Constant  Value=0
  const3 : Constant  Value=2
  output : Outport  OutputWhenDisabled=reset  InitialOutput=[0]
  wires:
  const/1 -> Interpreted MATLAB Function/1
  Interpreted MATLAB Function/1 -> Add/1, Product/2
  const1/1 -> Add/2
  Add/1 -> Product1/1
  Product/1 -> Switch1/3
  Switch1/1 -> Switch2/1
  Bus Selector/2 -> Switch1/2  "<out_neg>"
  Bus Selector/1 -> Product/1, Product1/2  "<out_amplitude>"
  konf/1 -> Bus Selector/1
  Switch2/1 -> output/1
  flank/1 -> Switch2/2
  const2/1 -> Switch2/3
  const3/1 -> Product2/1
  Product1/1 -> Product2/2
  Product2/1 -> Switch1/1

== system SensorFaultInj/FIM_Muster/Fault Injection Modul/AFI - additive faults injection/spike ==
  konf : Inport
  flank : Inport  Port=2
  xml_id : Inport  Port=3
  Enable : EnablePort  StatesWhenEnabling=reset
  Bus Selector : BusSelector  OutputSignals=spi_length,spi_factor
  Constant : Constant
  Constant1 : Constant  Value=0
  Constant2 : Constant  Value=7  OutDataTypeStr=single
  Discrete-Time Integrator : DiscreteIntegrator  gainval=1  ExternalReset=falling  SampleTime=SampleTime  ICPrevOutput=DiscIntNeverNeededParam  ICPrevScaledInput=DiscIntNeverNeededParam
  Product : Product
  Switch : Switch  Threshold=1
  ex_sfun_spikefcn : S-Function  FunctionName=ex_sfun_spikefcn  EnableBusSupport=off  mask(Legacy Function){SFunctionSpec=double y1 = spike_fcn(single u1, single u2, double u3, double u4), ShowSpec=on}
      mask prompts: ShowSpec "Display function specification"
      mask help:
      | This block allows you to call the legacy functions specified by the following Legacy Code Tool definition:
      | def.SFunctionName = 'ex_sfun_spikefcn';
      | def.OutputFcnSpec = 'double y1 = spike_fcn(single u1, single u2, double u3, double u4)';
      | def.HeaderFiles = {'spike_fcn.hpp'};
      | def.SourceFiles = {'spike_fcn.cpp'};
      | def.Options.language = 'C++';
      mask Help: <p>This block was generated automatically by the Legacy Code Tool. For detailed help on this tool, call<a href="matlab:legacy_code('help')"> legacy_code('help')</a>.</p>
      mask Callback ShowSpec:
      | if strcmp(get_param(gcbh, 'ShowSpec'), 'on')
      |   set_param(gcbh, 'MaskDisplay', sprintf('fprintf(''%s'');', get_param(gcbh, 'SFunctionSpec')));
      | else
      |   set_param(gcbh, 'MaskDisplay', sprintf('fprintf(''%s'');', get_param(gcbh, 'FunctionName')));
      | end
      mask Display: fprintf('double y1 = spike_fcn(single u1, single u2, double u3, double u4)');
  output : Outport  OutputWhenDisabled=reset  InitialOutput=[0]
  wires:
  Constant1/1 -> Switch/3
  Switch/1 -> Discrete-Time Integrator/1
  flank/1 -> Discrete-Time Integrator/2, Switch/2
  Constant/1 -> Switch/1
  Discrete-Time Integrator/1 -> ex_sfun_spikefcn/4
  xml_id/1 -> ex_sfun_spikefcn/2
  Constant2/1 -> ex_sfun_spikefcn/1
  Product/1 -> output/1
  konf/1 -> Bus Selector/1
  Bus Selector/1 -> ex_sfun_spikefcn/3  "<spi_length>"
  ex_sfun_spikefcn/1 -> Product/2
  Bus Selector/2 -> Product/1  "<spi_factor>"

== system SensorFaultInj/FIM_Muster/Fault Injection Modul/AFI - additive faults injection/stuck at x generation ==
  input : Inport
  konf : Inport  Port=2
  flank : Inport  Port=3
  enable : Inport  Port=4
  Bus Selector : BusSelector  OutputSignals=stx_min,stx_max
  Switch1 : Switch  Threshold=1
  Switch2 : Switch  Threshold=1
  Triggered Subsystem1 : Subsystem  TreatAsAtomicUnit=on
  output : Outport
  wires:
  konf/1 -> Bus Selector/1
  input/1 -> Switch2/3, Switch1/3, Triggered Subsystem1/1("In1 ")
  flank/1 -> Switch1/2, Triggered Subsystem1/Trigger
  Triggered Subsystem1/1(Out1) -> Switch1/1
  enable/1 -> Switch2/2
  Switch1/1 -> Switch2/1
  Switch2/1 -> output/1

== system SensorFaultInj/FIM_Muster/Fault Injection Modul/AFI - additive faults injection/stuck at x generation1 ==
  input : Inport
  konf : Inport  Port=2
  flank : Inport  Port=3
  enable : Inport  Port=4
  Bus Selector : BusSelector  OutputSignals=stx_min,stx_max
  Switch1 : Switch  Threshold=1
  Switch2 : Switch  Threshold=1
  Triggered Subsystem : Subsystem  TreatAsAtomicUnit=on
  output : Outport
  wires:
  konf/1 -> Bus Selector/1
  Bus Selector/2 -> Triggered Subsystem/2(bottom border)  "<stx_max>"
  Bus Selector/1 -> Triggered Subsystem/1(top border)  "<stx_min>"
  input/1 -> Switch2/3, Switch1/3
  flank/1 -> Triggered Subsystem/Trigger, Switch1/2
  Triggered Subsystem/1(Out1) -> Switch1/1
  enable/1 -> Switch2/2
  Switch1/1 -> Switch2/1
  Switch2/1 -> output/1

== system SensorFaultInj/FIM_Muster/Fault Injection Modul/AFI - additive faults injection/stuck at zero generation ==
  input : Inport
  flank : Inport  Port=2
  enable : Inport  Port=3
  Constant : Constant  Value=0
  Switch : Switch  Threshold=1
  Switch1 : Switch  Threshold=1
  output : Outport
  wires:
  Switch/1 -> Switch1/1
  Switch1/1 -> output/1
  enable/1 -> Switch1/2
  input/1 -> Switch/3, Switch1/3
  Constant/1 -> Switch/1
  flank/1 -> Switch/2

== system SensorFaultInj/FIM_Muster/Fault Injection Modul/FFI - functional fault injection/const delay  ==
  input : Inport
  konf : Inport  Port=2
  enable : Inport  Port=3
  Switch : Switch  Criteria=u2 ~= 0
  Variable Time Delay : VariableTransportDelay  MaximumDelay=10
  Zero-Order Hold : ZeroOrderHold  SampleTime=SampleTime
  output1 : Outport  OutputWhenDisabled=reset  InitialOutput=[0]
  delay : Outport  Port=2  OutputWhenDisabled=reset  InitialOutput=[0]
  wires:
  input/1 -> Switch/3, Variable Time Delay/1
  Switch/1 -> output1/1
  enable/1 -> Switch/2
  konf/1 -> delay/1, Variable Time Delay/2
  Variable Time Delay/1 -> Zero-Order Hold/1
  Zero-Order Hold/1 -> Switch/1

== system SensorFaultInj/FIM_Muster/Fault Injection Modul/FFI - functional fault injection/saturation ==
  input : Inport
  "konf " : Inport  Port=2
  enable : Inport  Port=3
  Demux1 : Demux  Outputs=2
  Divide : Product  Inputs=*/
  Divide1 : Product  Inputs=*/
  Switch : Switch  Criteria=u2 ~= 0
  Switch1 : Switch  Threshold=1
  Switch2 : Switch  Threshold=1
  output : Outport  OutputWhenDisabled=reset  InitialOutput=[0]
  wires:
  input/1 -> Switch/3, Switch1/3, Divide/1
  Divide/1 -> Switch1/2
  Switch1/1 -> Divide1/1, Switch2/3
  Divide1/1 -> Switch2/2
  Switch2/1 -> Switch/1
  Demux1/1 -> Switch1/1, Divide/2
  Demux1/2 -> Switch2/1, Divide1/2
  "konf "/1 -> Demux1/1
  Switch/1 -> output/1
  enable/1 -> Switch/2

== system SensorFaultInj/FIM_Muster/Fault Injection Modul/FFI - functional fault injection/time correlated delay  ==
  input : Inport
  konf : Inport  Port=2
  enable : Inport  Port=3
  xml id : Inport  Port=4
  Gain : Gain  Gain=-1
  Product : Product
  Product1 : Product
  Switch : Switch  Criteria=u2 ~= 0
  Switch1 : Switch  Criteria=u2 > Threshold
  Variable Time Delay : VariableTransportDelay  MaximumDelay=10  ZeroDelay=on
  Zero-Order Hold : ZeroOrderHold  SampleTime=SampleTime
  amplitude : Constant
  const : Constant  Value=0
  expr_parser : Subsystem
  output1 : Outport  OutputWhenDisabled=reset  InitialOutput=[0]
  delay : Outport  Port=2  OutputWhenDisabled=reset  InitialOutput=[0]
  wires:
  input/1 -> Switch/3, Variable Time Delay/1
  Switch/1 -> output1/1
  enable/1 -> Switch/2
  konf/1 -> Product/2
  Switch1/1 -> delay/1, Variable Time Delay/2
  Product1/1 -> Product/1
  amplitude/1 -> Product1/1
  expr_parser/1(corelation value) -> Product1/2
  xml id/1 -> expr_parser/1(xml id)
  Variable Time Delay/1 -> Zero-Order Hold/1
  Zero-Order Hold/1 -> Switch/1
  Gain/1 -> Switch1/2
  const/1 -> Switch1/1
  Product/1 -> Switch1/3, Gain/1

== system SensorFaultInj/FIM_Muster/Fault Injection Modul/MFI - multiplicative fault injection/time correlated noise ==
  konf : Inport
  flank : Inport  Port=2
  xml id : Inport  Port=3
  Enable : EnablePort
  Product2 : Product  Inputs=3
  Scope : Scope
      settings: SaveName=ScopeData21
  Switch1 : Switch  Threshold=1
  expr_parser1 : Subsystem
  pdf_parser : Subsystem
  zero : Constant  Value=0
  output : Outport  OutputWhenDisabled=reset  InitialOutput=[0]
  wires:
  flank/1 -> Switch1/2
  Switch1/1 -> output/1
  zero/1 -> Switch1/3
  expr_parser1/1(corelation value) -> Product2/1
  xml id/1 -> pdf_parser/1(xml id), expr_parser1/1(xml id)
  konf/1 -> Product2/3
  pdf_parser/1(distr value) -> Product2/2
  Product2/1 -> Switch1/1, Scope/1

== system SensorFaultInj/FIM_Muster/Fault Injection Modul/MFI - multiplicative fault injection/time correlated offset ==
  konf : Inport
  xml id : Inport  Port=2
  Enable : EnablePort
  Product : Product
  Scope : Scope  NumInputPorts=2
      settings: TimeRange=10  YMin=-5~-5  YMax=5~5  SaveName=ScopeData22
  expr_parser : Subsystem
  output : Outport  OutputWhenDisabled=reset  InitialOutput=[0]
  wires:
  Product/1 -> Scope/1, output/1
  expr_parser/1(corelation value) -> Product/2, Scope/2
  konf/1 -> Product/1
  xml id/1 -> expr_parser/1(xml id)

== system SensorFaultInj/FIM_Muster/Fault Injection Modul/MFI - multiplicative fault injection/value correlated noise ==
  input : Inport
  konf : Inport  Port=2
  flank : Inport  Port=3
  xml_id : Inport  Port=4
  Enable : EnablePort
  Product1 : Product  RndMeth=Zero
  Product2 : Product  RndMeth=Zero
  Switch : Switch  Threshold=1
  pdf_parser : Subsystem
  zero : Constant  Value=0
  output : Outport  OutputWhenDisabled=reset  InitialOutput=[0]
  wires:
  zero/1 -> Switch/3
  Switch/1 -> output/1
  input/1 -> Product2/1
  pdf_parser/1(distr value) -> Product1/2
  Product2/1 -> Product1/1
  Product1/1 -> Switch/1
  flank/1 -> Switch/2
  xml_id/1 -> pdf_parser/1(xml id)
  konf/1 -> Product2/2

== system SensorFaultInj/FIM_Muster/Fault Injection Modul/MFI - multiplicative fault injection/value correlated offset ==
  input : Inport
  konf : Inport  Port=2
  Enable : EnablePort
  Product : Product  RndMeth=Zero
  Subtract : Sum  Inputs=+-
  output : Outport  OutputWhenDisabled=reset  InitialOutput=[0]
  wires:
  input/1 -> Subtract/1, Product/1
  konf/1 -> Product/2
  Product/1 -> Subtract/2
  Subtract/1 -> output/1

== system SensorFaultInj/FIM_Muster/Parser Modul/Fault Parameter Parser/Enabled Subsystem ==
  In1 : Inport
  Enable : EnablePort
  Bus Creator : BusCreator  Inputs=13
  param_fcn id 0 : Subsystem
  param_fcn id 1 : Subsystem
  param_fcn id 10 : Subsystem
  param_fcn id 11 : Subsystem
  param_fcn id 12 : Subsystem
  param_fcn id 2 : Subsystem
  param_fcn id 3 : Subsystem
  param_fcn id 4 : Subsystem
  param_fcn id 5 : Subsystem
  param_fcn id 6 : Subsystem
  param_fcn id 7 : Subsystem
  param_fcn id 8 : Subsystem
  param_fcn id 9 : Subsystem
  Out1 : Outport  LockScale=on
  wires:
  Bus Creator/1 -> Out1/1  "parameter_bus"
  In1/1 -> param_fcn id 1/1(In1), param_fcn id 3/1(In1), param_fcn id 5/1(In1), param_fcn id 6/1(In1), param_fcn id 7/1(In1), param_fcn id 8/1(In1), param_fcn id 9/1(In1), param_fcn id 10/1(In1), param_fcn id 12/1(In1), param_fcn id 11/1(In1), param_fcn id 4/1(In1), param_fcn id 2/1(In1), param_fcn id 0/1(In1)
  param_fcn id 8/1(Out1) -> Bus Creator/9
  param_fcn id 4/1(Out1) -> Bus Creator/5
  param_fcn id 6/1(Out1) -> Bus Creator/7
  param_fcn id 2/1(Out1) -> Bus Creator/3
  param_fcn id 1/1(Out1) -> Bus Creator/2
  param_fcn id 3/1(Out1) -> Bus Creator/4
  param_fcn id 7/1(Out1) -> Bus Creator/8
  param_fcn id 0/1(Out1) -> Bus Creator/1
  param_fcn id 5/1(Out1) -> Bus Creator/6
  param_fcn id 11/1(Out1) -> Bus Creator/12
  param_fcn id 12/1(Out1) -> Bus Creator/13
  param_fcn id 9/1(Out1) -> Bus Creator/10
  param_fcn id 10/1(Out1) -> Bus Creator/11

== system SensorFaultInj/FIM_Muster/Parser Modul/Occurence Parser /Enabled Subsystem ==
  In1 : Inport
  Enable : EnablePort
  Bus Creator : BusCreator  Inputs=7
  occurnce parser fault id 2 : Subsystem
  occurnce parser fault id 3 : Subsystem
  occurnce parser fault id 5 : Subsystem
  occurnce parser fault id 6 : Subsystem
  occurnce parser fault id 7 : Subsystem
  occurnce parser fault id 8 : Subsystem
  occurnce parser fault id 9 : Subsystem
  Out1 : Outport
  wires:
  occurnce parser fault id 8/1(Out1) -> Bus Creator/6
  occurnce parser fault id 5/1(Out1) -> Bus Creator/3
  occurnce parser fault id 7/1(Out1) -> Bus Creator/5
  occurnce parser fault id 6/1(Out1) -> Bus Creator/4
  occurnce parser fault id 2/1(Out1) -> Bus Creator/1
  occurnce parser fault id 3/1(Out1) -> Bus Creator/2
  occurnce parser fault id 9/1(Out1) -> Bus Creator/7
  Bus Creator/1 -> Out1/1  "occurrence_bus"
  In1/1 -> occurnce parser fault id 3/1(In1), occurnce parser fault id 5/1(In1), occurnce parser fault id 6/1(In1), occurnce parser fault id 7/1(In1), occurnce parser fault id 8/1(In1), occurnce parser fault id 9/1(In1), occurnce parser fault id 2/1(In1)

== system SensorFaultInj/FIM_Muster/Parser Modul/Schedule Parser and Generator /schedule_fcn id 0 ==
  In1 : Inport
  Discrete-Time Integrator : DiscreteIntegrator  SampleTime=-1  ICPrevOutput=DiscIntNeverNeededParam  ICPrevScaledInput=DiscIntNeverNeededParam
  Scope1 : Scope  NumInputPorts=2
      settings: YMin=-5~-5  YMax=5~5  SaveName=ScopeData25
  SimLength : Constant  Value=SimLength
  ex_sfun_schedulefcn1 : S-Function  FunctionName=ex_sfun_schedulefcn  EnableBusSupport=off  mask(Legacy Function){SFunctionSpec=single y1 = schedule_fcn(double u1, double u2, single u3, single u4), ShowSpec=on}
      mask prompts: ShowSpec "Display function specification"
      mask help:
      | This block allows you to call the legacy functions specified by the following Legacy Code Tool definition:
      | def.SFunctionName = 'ex_sfun_schedulefcn';
      | def.OutputFcnSpec = 'single y1 = schedule_fcn(double u1, double u2, single u3, single u4)';
      | def.HeaderFiles = {'schedule_fcn.hpp'};
      | def.SourceFiles = {'schedule_fcn.cpp'};
      | def.Options.language = 'C++';
      mask Help: <p>This block was generated automatically by the Legacy Code Tool. For detailed help on this tool, call<a href="matlab:legacy_code('help')"> legacy_code('help')</a>.</p>
      mask Callback ShowSpec:
      | if strcmp(get_param(gcbh, 'ShowSpec'), 'on')
      |   set_param(gcbh, 'MaskDisplay', sprintf('fprintf(''%s'');', get_param(gcbh, 'SFunctionSpec')));
      | else
      |   set_param(gcbh, 'MaskDisplay', sprintf('fprintf(''%s'');', get_param(gcbh, 'FunctionName')));
      | end
      mask Display: fprintf('single y1 = schedule_fcn(double u1, double u2, single u3, single u4)');
  "fault_id " : Constant  Value=0  OutDataTypeStr=single
  one : Constant
  output : Outport  OutputWhenDisabled=reset  InitialOutput=[0]
  wires:
  one/1 -> Discrete-Time Integrator/1
  Discrete-Time Integrator/1 -> ex_sfun_schedulefcn1/2, Scope1/2
  ex_sfun_schedulefcn1/1 -> Scope1/1, output/1  "vco_schedule"
  SimLength/1 -> ex_sfun_schedulefcn1/1
  "fault_id "/1 -> ex_sfun_schedulefcn1/3
  In1/1 -> ex_sfun_schedulefcn1/4
